simulink model "mdl1"  (R2013b)
settings: Solver=ode1  StartTime=0.0  StopTime=tSim  FixedStep=h  RelTol=1e-3
values from neighbouring files (symbols this model uses):
  y0 = 3    [test.m]
settings Model: Creator=JAR  LastModifiedBy=JAR

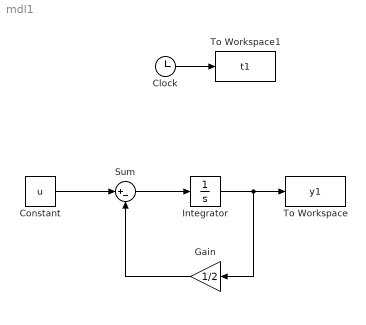
== system mdl1 ==
  Clock : Clock
  Constant : Constant  Value=u
  Gain : Gain  Gain=1/2
  Integrator : Integrator  InitialCondition=y0
  Sum : Sum  Inputs=|+-
  To Workspace : ToWorkspace  VariableName=y1  SampleTime=-1
  To Workspace1 : ToWorkspace  VariableName=t1  SampleTime=-1
  wires:
  Clock/1 -> To Workspace1/1
  Constant/1 -> Sum/1
  Integrator/1 -> Gain/1, To Workspace/1
  Sum/1 -> Integrator/1
  Gain/1 -> Sum/2
